simulink model "Demo_Microgrid_OP4510"  (R2017b)
settings: Solver=ode4  StartTime=0.0  StopTime=inf  FixedStep=sim.dt  RelTol=1e-3
values from neighbouring files (symbols this model uses):
  DS001_f0 = 50    [Script_Initialization.m]
  DS001_p0 = 500    [Script_Initialization.m]
  f0_vsi_2 = 50    [Script_Initialization.m]
  kp_vsi_2 = (f0_vsi_2/pmax_vsi_2)*3/1000    (= 7.5e-05)    [Script_Initialization.m]
  kq_vsi_1 = 1e-3    (= 0.001)    [Script_Initialization.m]
  kq_vsi_2 = 1e-3    (= 0.001)    [Script_Initialization.m]
  L_vsi_1 = 2e-3    (= 0.002)    [Script_Initialization.m]
  L_vsi_2 = 2e-3    (= 0.002)    [Script_Initialization.m]
  on_vsi_2 = 1    [Script_Initialization.m]
  p0_vsi_2 = 500    [Script_Initialization.m]
  phi0Deg_vsi_2 = phi0_vsi_2*180/pi    (= 45)    [Script_Initialization.m]
  q0_vsi_2 = 0    [Script_Initialization.m]
  R_vsi_1 = 1e-1    (= 0.1)    [Script_Initialization.m]
  R_vsi_2 = 1e-1    (= 0.1)    [Script_Initialization.m]
  tp_vsi_2 = 100e-3    (= 0.1)    [Script_Initialization.m]
  tq_vsi_1 = 10e-3    (= 0.01)    [Script_Initialization.m]
  tq_vsi_2 = 10e-3    (= 0.01)    [Script_Initialization.m]
  v0_vsi_2 = 340*sqrt(2)    [Script_Initialization.m]
undefined symbols (not defined in the file or in its folder): ld_1, sim, vsi
libraries: powerlib x22, powerlib_meascontrol x5, rtlab x2, xpcrtudplib x2, etargetslib x1, embdlinuxlib x1
settings Model: xpc_rtwmakecfg_data=_xpcnblib__xpcetherlib__xpcether8255xlib__xpcetherGbElib__xpciplib_  Creator=Edwin_Mora  LastModifiedBy=EINS_Admin
settings DebuggingCC: UnconnectedInputMsg=none  UnconnectedOutputMsg=none  UnconnectedLineMsg=none
settings ConfigComp: PSAutoStubLUT=on

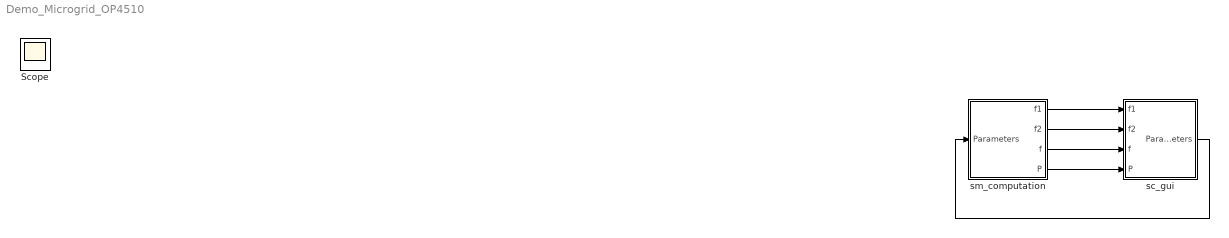
== system Demo_Microgrid_OP4510 ==
  sc_gui : Subsystem
  sm_computation : Subsystem
  Scope : Scope
  wires:
  sm_computation/1(f1) -> sc_gui/1(f1)
  sm_computation/2(f2) -> sc_gui/2(f2)
  sc_gui/1(Parameters) -> sm_computation/1(Parameters)
  sm_computation/3(f) -> sc_gui/3(f)
  sm_computation/4("P ") -> sc_gui/4(P)

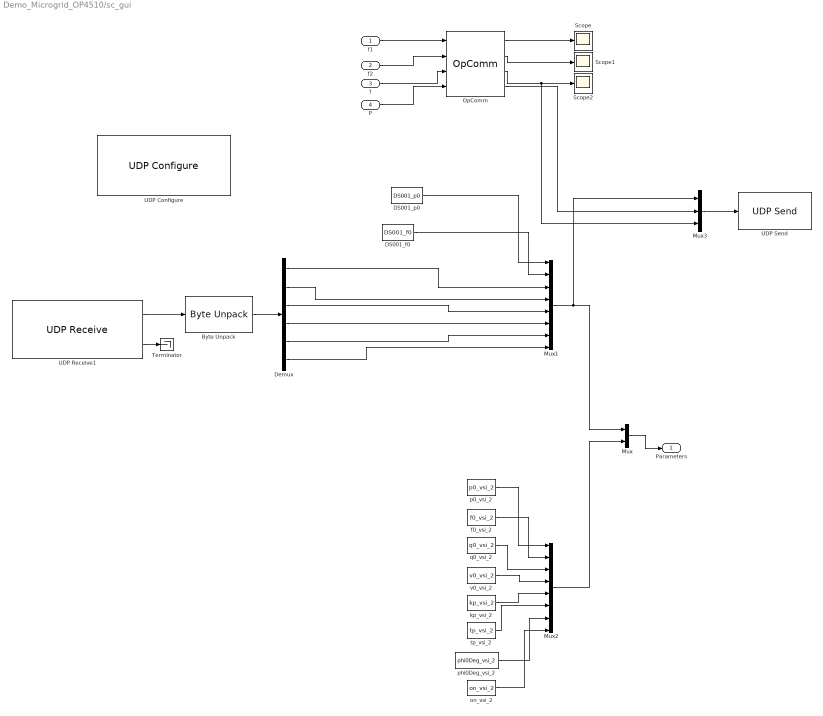
== system Demo_Microgrid_OP4510/sc_gui ==
  f1 : Inport
  f2 : Inport  Port=2
  f : Inport  Port=3
  P : Inport  Port=4
  Byte Unpack : etargetslib/Byte Unpack  dimensions={[6]}  datatypes={'double'}  byteAlign=1
  DS001_f0 : Constant  Value=DS001_f0
  DS001_p0 : Constant  Value=DS001_p0
  Demux : Demux  Outputs=6
  Mux : Mux  Inputs=2
  Mux1 : Mux  Inputs=8
  Mux2 : Mux  Inputs=8
  Mux3 : Mux  Inputs=3
  OpComm : rtlab/OpComm  nbport=4  groupe_acq=1  subsys_rate=0  st=0  Synchronization=on  Interpolation=on  Threshold=1.0  Missed_Data=off  Sim_Time=off  Samples=off  dynSigOut=off  from_console=0  warning_done=off  writeOpCommFile=off  Offset=off
  Scope : Scope
  Scope1 : Scope
  Scope2 : Scope
  Terminator : Terminator
  UDP Configure : xpcrtudplib/UDP Configure  Priority=-1  IpAddress=192.168.1.100  SubnetMask=255.255.255.0  Gateway=0.0.0.0  PciBus=[0]  PciSlot=[6]  PciFunction=0  ID=1  tune=0
      settings: SourceProductName=Simulink Real-Time  SourceProductBaseCode=XP
  UDP Receive1 : xpcrtudplib/UDP Receive  ipAddressVal=192.168.1.100  localPort=8002  rcvWidth=48  rcvFmAny=on  fmAddress=0.0.0.0  maxUDPQueue=8  sampleTime=-1
      settings: SourceProductName=Simulink Real-Time
  UDP Send : embdlinuxlib/UDP Send  remoteURL='192.168.1.11'  remotePort=8001  localURL='255.255.255.255'  localPortSource=Automatically determine  localPort=-1  sampletime=-1  blockPlatform=Raspberry Pi  separateLengthPort=0
      settings: SourceProductName=Simulink Support Package for Raspberry Pi Hardware  SourceProductBaseCode=RASPPI
  f0_vsi_2 : Constant  Value=f0_vsi_2
  kp_vsi_2 : Constant  Value=kp_vsi_2
  on_vsi_2 : Constant  Value=on_vsi_2
  p0_vsi_2 : Constant  Value=p0_vsi_2
  phi0Deg_vsi_2 : Constant  Value=phi0Deg_vsi_2
  q0_vsi_2 : Constant  Value=q0_vsi_2
  tp_vsi_2 : Constant  Value=tp_vsi_2
  v0_vsi_2 : Constant  Value=v0_vsi_2
  Parameters : Outport
  wires:
  f1/1 -> OpComm/1
  OpComm/1 -> Scope/1
  Mux/1 -> Parameters/1
  DS001_p0/1 -> Mux1/1
  DS001_f0/1 -> Mux1/2
  Mux1/1 -> Mux3/1, Mux/1
  f0_vsi_2/1 -> Mux2/2
  p0_vsi_2/1 -> Mux2/1
  on_vsi_2/1 -> Mux2/8
  q0_vsi_2/1 -> Mux2/3
  kp_vsi_2/1 -> Mux2/5
  tp_vsi_2/1 -> Mux2/6
  phi0Deg_vsi_2/1 -> Mux2/7
  v0_vsi_2/1 -> Mux2/4
  Mux2/1 -> Mux/2
  f/1 -> OpComm/3
  OpComm/3 -> Mux3/3, Scope2/1
  f2/1 -> OpComm/2
  OpComm/2 -> Scope1/1
  Mux3/1 -> UDP Send/1
  P/1 -> OpComm/4
  OpComm/4 -> Mux3/2
  UDP Receive1/1 -> Byte Unpack/1
  Demux/1 -> Mux1/3
  Demux/2 -> Mux1/4
  Demux/3 -> Mux1/5
  Demux/4 -> Mux1/6
  Demux/5 -> Mux1/7
  Demux/6 -> Mux1/8
  Byte Unpack/1 -> Demux/1
  UDP Receive1/2 -> Terminator/1

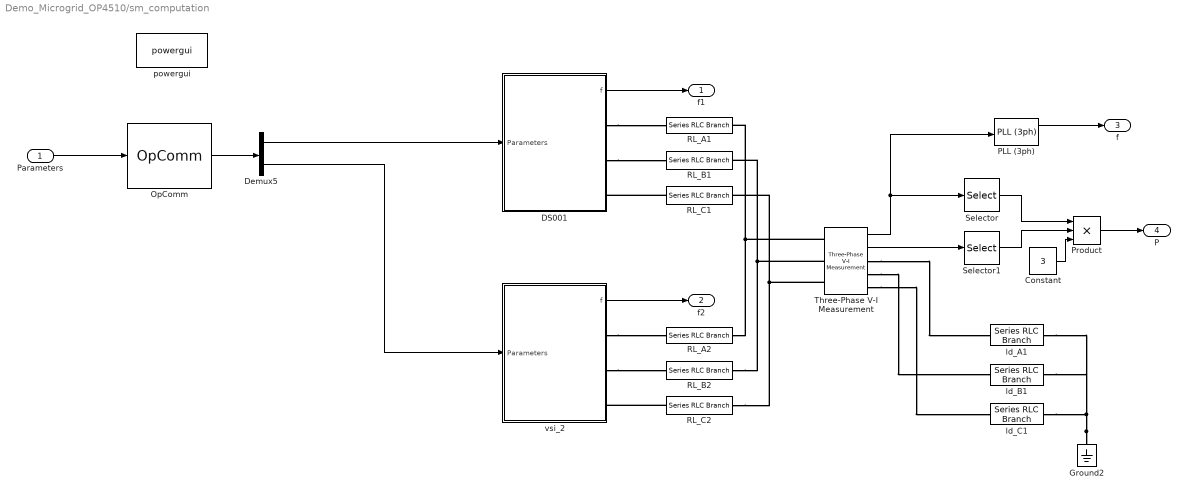
== system Demo_Microgrid_OP4510/sm_computation ==
  Parameters : Inport
  Constant : Constant  Value=3
  DS001 : Subsystem
  Demux5 : Demux  Outputs=2
  Ground2 : powerlib/Elements/Ground  LConnTagsString=a
  OpComm : rtlab/OpComm  nbport=1  groupe_acq=1  subsys_rate=sim.dt  st=0  Synchronization=on  Interpolation=on  Threshold=1.0  Missed_Data=off  Sim_Time=off  Samples=off  dynSigOut=off  from_console=1  warning_done=off  writeOpCommFile=off  Offset=off
  PLL (3ph) : powerlib_meascontrol/PLL/PLL (3ph)  Fmin=45  Par_Init=[0, 50]  ParK=[180, 3200, 1]  TcD=1e-4  MaxRateChangeFreq=12  FilterCutOffFreq=25  Ts=0  AGC=on
  Product : Product  Inputs=3
  RL_A1 : powerlib/Elements/Series RLC Branch  LConnTagsString=__new0  RConnTagsString=__new0  BranchType=RL  Resistance=R_vsi_1  Inductance=L_vsi_1  SetiL0=on  InitialCurrent=0  Capacitance=1e-6  Setx0=off  InitialVoltage=0  Measurements=None
  RL_A2 : powerlib/Elements/Series RLC Branch  LConnTagsString=__new0  RConnTagsString=__new0  BranchType=RL  Resistance=R_vsi_2  Inductance=L_vsi_2  SetiL0=on  InitialCurrent=0  Capacitance=1e-6  Setx0=off  InitialVoltage=0  Measurements=None
  RL_B1 : powerlib/Elements/Series RLC Branch  LConnTagsString=__new0  RConnTagsString=__new0  BranchType=RL  Resistance=R_vsi_1  Inductance=L_vsi_1  SetiL0=on  InitialCurrent=0  Capacitance=1e-6  Setx0=off  InitialVoltage=0  Measurements=None
  RL_B2 : powerlib/Elements/Series RLC Branch  LConnTagsString=__new0  RConnTagsString=__new0  BranchType=RL  Resistance=R_vsi_2  Inductance=L_vsi_2  SetiL0=on  InitialCurrent=0  Capacitance=1e-6  Setx0=off  InitialVoltage=0  Measurements=None
  RL_C1 : powerlib/Elements/Series RLC Branch  LConnTagsString=__new0  RConnTagsString=__new0  BranchType=RL  Resistance=R_vsi_1  Inductance=L_vsi_1  SetiL0=on  InitialCurrent=0  Capacitance=1e-6  Setx0=off  InitialVoltage=0  Measurements=None
  RL_C2 : powerlib/Elements/Series RLC Branch  LConnTagsString=__new0  RConnTagsString=__new0  BranchType=RL  Resistance=R_vsi_2  Inductance=L_vsi_2  SetiL0=on  InitialCurrent=0  Capacitance=1e-6  Setx0=off  InitialVoltage=0  Measurements=None
  Selector : Selector  InputPortWidth=3  IndexOptions=Index vector (dialog)  Indices=[1]  OutputSizes=1
  Selector1 : Selector  InputPortWidth=3  IndexOptions=Index vector (dialog)  Indices=[1]  OutputSizes=1
  Three-Phase V-I Measurement : powerlib/Measurements/Three-Phase V-I Measurement  VoltageMeasurement=phase-to-ground  SetLabelV=off  LabelV=Vabc  Vpu=off  VpuLL=off  CurrentMeasurement=yes  SetLabelI=off  LabelI=Iabc  Ipu=off  Pbase=100e6  Vbase=500e3  OutputType=Complex  PhasorSimulation=off  PSBequivalent=0
  ld_A1 : powerlib/Elements/Series RLC Branch  LConnTagsString=__new0  RConnTagsString=__new0  BranchType=R  Resistance=ld_1.R  Inductance=1e-3  SetiL0=off  InitialCurrent=0  Capacitance=1e-6  Setx0=off  InitialVoltage=0  Measurements=None
  ld_B1 : powerlib/Elements/Series RLC Branch  LConnTagsString=__new0  RConnTagsString=__new0  BranchType=R  Resistance=ld_1.R  Inductance=1e-3  SetiL0=off  InitialCurrent=0  Capacitance=1e-6  Setx0=off  InitialVoltage=0  Measurements=None
  ld_C1 : powerlib/Elements/Series RLC Branch  LConnTagsString=__new0  RConnTagsString=__new0  BranchType=R  Resistance=ld_1.R  Inductance=1e-3  SetiL0=off  InitialCurrent=0  Capacitance=1e-6  Setx0=off  InitialVoltage=0  Measurements=None
  powergui : powerlib/powergui  Priority=1  SimulationMode=Discrete  SampleTime=sim.dt  frequency=50  Iterations=50  frequencyindice=0  Pbase=100e6  ErrMax=1e-4  UnitsV=kV  UnitsW=MW  buscounter=0  FunctionMessages=off  echomessages=off  EnableUseOfTLC=off  CurrentSourceSwitches=off  DisableSnubberDevices=off  DisableRonSwitches=off  DisableVfSwitches=off  DisplayEquations=off  SolverType=Tustin/Backward Euler (TBE)  Interpol=off  ExternalGateDelay=off  methode=off  Ts=100  x0status=blocks  SPID=on  SwTol=0  HookPort=off  RestoreLinks=warning  ResistiveCurrentMeasurement=off  Frange=[0:2:500]  Ylog=off  Xlog=on  ShowGrid=off  save=off  variable=ZData  structure=0  ZoomFFT=off  StartTime=0.0  cycles=1  DisplayStyle=1  fundamental=60  FreqAxis=off  MaxFrequency=1000  frequencyindicesteady=1  RmsSteady=1  display=off
  vsi_2 : Subsystem
  f1 : Outport
  f2 : Outport  Port=2
  f : Outport  Port=3
  "P " : Outport  Port=4
  wires:
  OpComm/1 -> Demux5/1
  Demux5/1 -> DS001/1(Parameters)
  DS001/1(f) -> f1/1
  vsi_2/1(f) -> f2/1
  Demux5/2 -> vsi_2/1(Parameters)
  Parameters/1 -> OpComm/1
  PLL (3ph)/1 -> f/1
  Three-Phase V-I Measurement/1 -> Selector/1, PLL (3ph)/1
  Product/1 -> "P "/1
  Three-Phase V-I Measurement/2 -> Selector1/1
  Selector/1 -> Product/1
  Selector1/1 -> Product/2
  Constant/1 -> Product/3
  connections:
  Ground2/LConn1 -- ld_A1/RConn1 -- ld_B1/RConn1 -- ld_C1/RConn1
  DS001/RConn1 -- RL_A1/LConn1
  DS001/RConn2 -- RL_B1/LConn1
  RL_C1/LConn1 -- DS001/RConn3
  vsi_2/RConn1 -- RL_A2/LConn1
  vsi_2/RConn2 -- RL_B2/LConn1
  RL_C2/LConn1 -- vsi_2/RConn3
  RL_A2/RConn1 -- RL_A1/RConn1 -- Three-Phase V-I Measurement/LConn1
  RL_B2/RConn1 -- Three-Phase V-I Measurement/LConn2 -- RL_B1/RConn1
  RL_C2/RConn1 -- Three-Phase V-I Measurement/LConn3 -- RL_C1/RConn1
  Three-Phase V-I Measurement/RConn1 -- ld_A1/LConn1
  Three-Phase V-I Measurement/RConn2 -- ld_B1/LConn1
  Three-Phase V-I Measurement/RConn3 -- ld_C1/LConn1

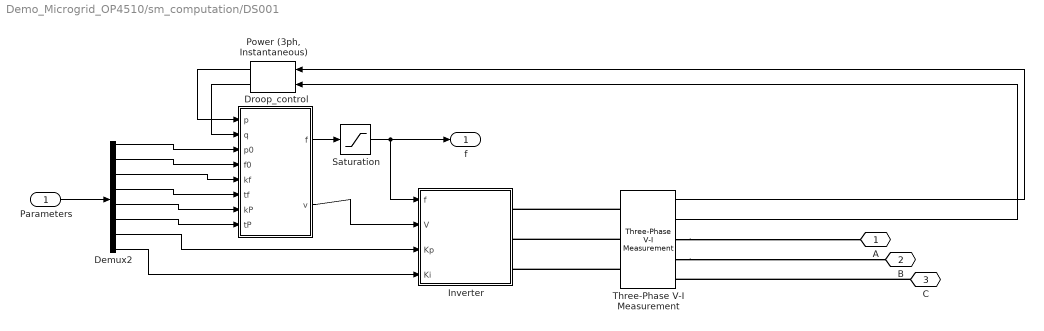
== system Demo_Microgrid_OP4510/sm_computation/DS001 ==
  Parameters : Inport
  Demux2 : Demux  Outputs=8
  Droop_control : Subsystem
  Inverter : Subsystem
  "Power (3ph, Instantaneous)" : powerlib_meascontrol/Measurements/Power (3ph, Instantaneous)
      settings: SourceProductName=Simscape Power Systems
  Saturation : Saturate  UpperLimit=inf  LowerLimit=0
  Three-Phase V-I Measurement : powerlib/Measurements/Three-Phase V-I Measurement  VoltageMeasurement=phase-to-ground  SetLabelV=off  LabelV=Vabc  Vpu=off  VpuLL=off  CurrentMeasurement=yes  SetLabelI=off  LabelI=Iabc  Ipu=off  Pbase=100e6  Vbase=500e3  OutputType=Complex  PhasorSimulation=off  PSBequivalent=0
  A : PMIOPort  Port=1  Side=Right
  B : PMIOPort  Port=2  Side=Right
  C : PMIOPort  Port=3  Side=Right
  f : Outport
  wires:
  Parameters/1 -> Demux2/1
  Demux2/2 -> Droop_control/4(f0)
  Droop_control/2(v) -> Inverter/2(V)
  Demux2/4 -> Droop_control/6(tf)
  Demux2/3 -> Droop_control/5(kf)
  Demux2/6 -> Droop_control/8(tP)
  Demux2/7 -> Inverter/3(Kp)
  Demux2/5 -> Droop_control/7(kP)
  Demux2/1 -> Droop_control/3(p0)
  Saturation/1 -> f/1, Inverter/1(f)
  "Power (3ph, Instantaneous)"/2 -> Droop_control/2(q)
  Three-Phase V-I Measurement/2 -> "Power (3ph, Instantaneous)"/2
  Droop_control/1(f) -> Saturation/1
  "Power (3ph, Instantaneous)"/1 -> Droop_control/1(p)
  Three-Phase V-I Measurement/1 -> "Power (3ph, Instantaneous)"/1
  Demux2/8 -> Inverter/4(Ki)
  connections:
  Three-Phase V-I Measurement/RConn2 -- B/RConn1
  Three-Phase V-I Measurement/LConn1 -- Inverter/RConn1
  Three-Phase V-I Measurement/LConn2 -- Inverter/RConn2
  Three-Phase V-I Measurement/LConn3 -- Inverter/RConn3
  Three-Phase V-I Measurement/RConn1 -- A/RConn1
  C/RConn1 -- Three-Phase V-I Measurement/RConn3

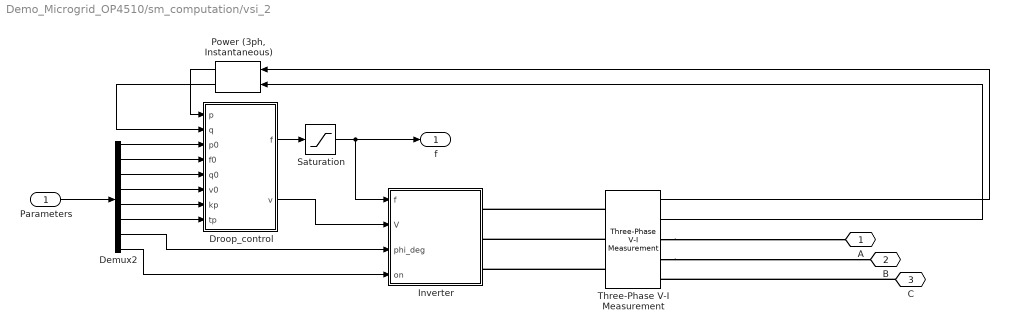
== system Demo_Microgrid_OP4510/sm_computation/vsi_2 ==
  Parameters : Inport
  Demux2 : Demux  Outputs=8
  Droop_control : Subsystem
  Inverter : Subsystem
  "Power (3ph, Instantaneous)" : powerlib_meascontrol/Measurements/Power (3ph, Instantaneous)
      settings: SourceProductName=Simscape Power Systems
  Saturation : Saturate  UpperLimit=inf  LowerLimit=0
  Three-Phase V-I Measurement : powerlib/Measurements/Three-Phase V-I Measurement  VoltageMeasurement=phase-to-ground  SetLabelV=off  LabelV=Vabc  Vpu=off  VpuLL=off  CurrentMeasurement=yes  SetLabelI=off  LabelI=Iabc  Ipu=off  Pbase=100e6  Vbase=500e3  OutputType=Complex  PhasorSimulation=off  PSBequivalent=0
  A : PMIOPort  Port=1  Side=Right
  B : PMIOPort  Port=2  Side=Right
  C : PMIOPort  Port=3  Side=Right
  f : Outport
  wires:
  Demux2/2 -> Droop_control/4(f0)
  Droop_control/2(v) -> Inverter/2(V)
  Demux2/4 -> Droop_control/6(v0)
  Demux2/3 -> Droop_control/5(q0)
  Demux2/6 -> Droop_control/8(tp)
  Parameters/1 -> Demux2/1
  Demux2/5 -> Droop_control/7(kp)
  Demux2/1 -> Droop_control/3(p0)
  Saturation/1 -> f/1, Inverter/1(f)
  "Power (3ph, Instantaneous)"/2 -> Droop_control/2(q)
  Three-Phase V-I Measurement/2 -> "Power (3ph, Instantaneous)"/2
  Droop_control/1(f) -> Saturation/1
  "Power (3ph, Instantaneous)"/1 -> Droop_control/1(p)
  Three-Phase V-I Measurement/1 -> "Power (3ph, Instantaneous)"/1
  Demux2/7 -> Inverter/3(phi_deg)
  Demux2/8 -> Inverter/4(on)
  connections:
  Three-Phase V-I Measurement/RConn2 -- B/RConn1
  Three-Phase V-I Measurement/LConn1 -- Inverter/RConn1
  Three-Phase V-I Measurement/LConn2 -- Inverter/RConn2
  Three-Phase V-I Measurement/LConn3 -- Inverter/RConn3
  Three-Phase V-I Measurement/RConn1 -- A/RConn1
  C/RConn1 -- Three-Phase V-I Measurement/RConn3

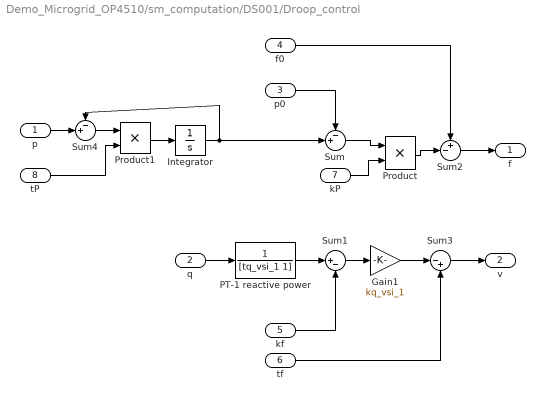
== system Demo_Microgrid_OP4510/sm_computation/DS001/Droop_control ==
  p : Inport
  q : Inport  Port=2
  p0 : Inport  Port=3
  f0 : Inport  Port=4
  kf : Inport  Port=5
  tf : Inport  Port=6
  kP : Inport  Port=7
  tP : Inport  Port=8
  Gain1 : Gain  Gain=kq_vsi_1
  Integrator : Integrator
  PT-1 reactive power : TransferFcn  Denominator=[tq_vsi_1 1]
  Product : Product
  Product1 : Product
  Sum : Sum  Inputs=-+|
  Sum1 : Sum  Inputs=|+-
  Sum2 : Sum  Inputs=+-|
  Sum3 : Sum  Inputs=|-+
  Sum4 : Sum  Inputs=-+|
  f : Outport
  v : Outport  Port=2
  wires:
  Product/1 -> Sum2/2
  Gain1/1 -> Sum3/1
  Sum1/1 -> Gain1/1
  Sum/1 -> Product/1
  Sum3/1 -> v/1
  Sum2/1 -> f/1
  PT-1 reactive power/1 -> Sum1/1
  q/1 -> PT-1 reactive power/1
  p0/1 -> Sum/1
  f0/1 -> Sum2/1
  kf/1 -> Sum1/2
  tf/1 -> Sum3/2
  kP/1 -> Product/2
  p/1 -> Sum4/2
  Sum4/1 -> Product1/1
  Product1/1 -> Integrator/1
  Integrator/1 -> Sum/2, Sum4/1
  tP/1 -> Product1/2

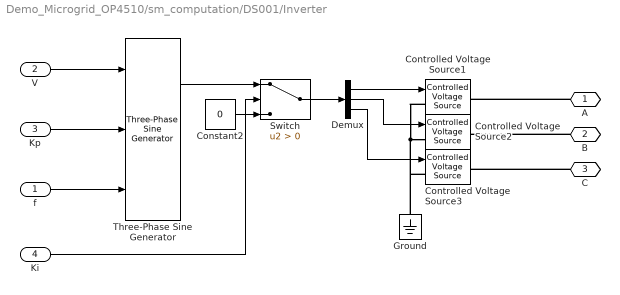
== system Demo_Microgrid_OP4510/sm_computation/DS001/Inverter ==
  f : Inport
  V : Inport  Port=2
  Kp : Inport  Port=3
  Ki : Inport  Port=4
  Constant2 : Constant  Value=0
  Controlled Voltage Source1 : powerlib/Electrical Sources/Controlled Voltage Source  Initialize=off  Source_Type=AC  Amplitude=vsi(1).v0  Phase=vsi(1).phi0*180/pi + 90  Frequency=vsi(1).f0  Measurements=None
  Controlled Voltage Source2 : powerlib/Electrical Sources/Controlled Voltage Source  Initialize=off  Source_Type=AC  Amplitude=vsi(1).v0  Phase=(vsi(1).phi0 - 2*pi/3)*180/pi + 90  Frequency=vsi(1).f0  Measurements=None
  Controlled Voltage Source3 : powerlib/Electrical Sources/Controlled Voltage Source  Initialize=off  Source_Type=AC  Amplitude=vsi(1).v0  Phase=(vsi(1).phi0 - 4*pi/3)*180/pi + 90  Frequency=vsi(1).f0  Measurements=None
  Demux : Demux  Outputs=3
  Ground : powerlib/Elements/Ground  LConnTagsString=a
  Switch : Switch  Criteria=u2 > Threshold
  Three-Phase Sine Generator : powerlib_meascontrol/Pulse & Signal Generators/Three-Phase Sine Generator  Ts=sim.dt
      settings: SourceProductName=Simscape Power Systems  SourceProductBaseCode=PS
  A : PMIOPort  Port=1  Side=Right
  B : PMIOPort  Port=2  Side=Right
  C : PMIOPort  Port=3  Side=Right
  wires:
  Ki/1 -> Switch/2
  f/1 -> Three-Phase Sine Generator/3
  Constant2/1 -> Switch/3
  Switch/1 -> Demux/1
  Three-Phase Sine Generator/1 -> Switch/1
  Demux/1 -> Controlled Voltage Source1/1
  V/1 -> Three-Phase Sine Generator/1
  Demux/3 -> Controlled Voltage Source3/1
  Kp/1 -> Three-Phase Sine Generator/2
  Demux/2 -> Controlled Voltage Source2/1
  connections:
  B/RConn1 -- Controlled Voltage Source2/RConn1
  A/RConn1 -- Controlled Voltage Source1/RConn1
  C/RConn1 -- Controlled Voltage Source3/RConn1
  Controlled Voltage Source1/LConn1 -- Ground/LConn1 -- Controlled Voltage Source3/LConn1 -- Controlled Voltage Source2/LConn1

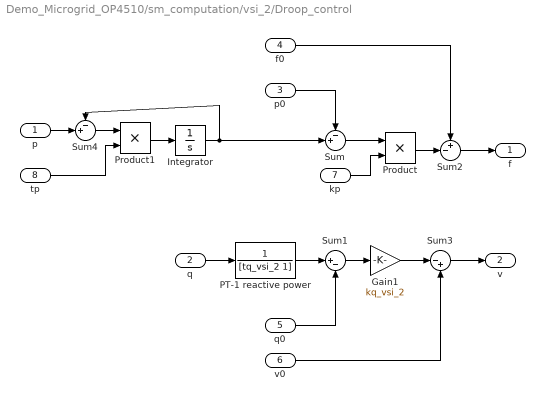
== system Demo_Microgrid_OP4510/sm_computation/vsi_2/Droop_control ==
  p : Inport
  q : Inport  Port=2
  p0 : Inport  Port=3
  f0 : Inport  Port=4
  q0 : Inport  Port=5
  v0 : Inport  Port=6
  kp : Inport  Port=7
  tp : Inport  Port=8
  Gain1 : Gain  Gain=kq_vsi_2
  Integrator : Integrator
  PT-1 reactive power : TransferFcn  Denominator=[tq_vsi_2 1]
  Product : Product
  Product1 : Product
  Sum : Sum  Inputs=-+|
  Sum1 : Sum  Inputs=|+-
  Sum2 : Sum  Inputs=+-|
  Sum3 : Sum  Inputs=|-+
  Sum4 : Sum  Inputs=-+|
  f : Outport
  v : Outport  Port=2
  wires:
  Product/1 -> Sum2/2
  Gain1/1 -> Sum3/1
  Sum1/1 -> Gain1/1
  Sum/1 -> Product/1
  Sum3/1 -> v/1
  Sum2/1 -> f/1
  PT-1 reactive power/1 -> Sum1/1
  q/1 -> PT-1 reactive power/1
  p0/1 -> Sum/1
  f0/1 -> Sum2/1
  q0/1 -> Sum1/2
  v0/1 -> Sum3/2
  kp/1 -> Product/2
  p/1 -> Sum4/2
  Sum4/1 -> Product1/1
  Product1/1 -> Integrator/1
  Integrator/1 -> Sum/2, Sum4/1
  tp/1 -> Product1/2

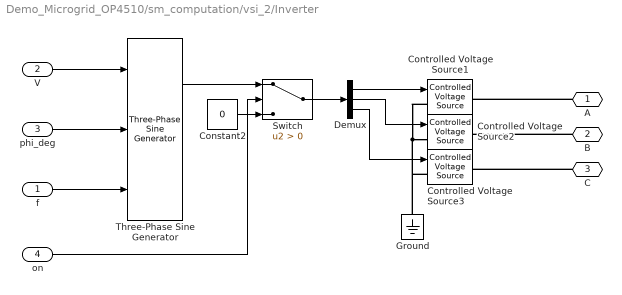
== system Demo_Microgrid_OP4510/sm_computation/vsi_2/Inverter ==
  f : Inport
  V : Inport  Port=2
  phi_deg : Inport  Port=3
  on : Inport  Port=4
  Constant2 : Constant  Value=0
  Controlled Voltage Source1 : powerlib/Electrical Sources/Controlled Voltage Source  Initialize=off  Source_Type=AC  Amplitude=vsi(1).v0  Phase=vsi(1).phi0*180/pi + 90  Frequency=vsi(1).f0  Measurements=None
  Controlled Voltage Source2 : powerlib/Electrical Sources/Controlled Voltage Source  Initialize=off  Source_Type=AC  Amplitude=vsi(1).v0  Phase=(vsi(1).phi0 - 2*pi/3)*180/pi + 90  Frequency=vsi(1).f0  Measurements=None
  Controlled Voltage Source3 : powerlib/Electrical Sources/Controlled Voltage Source  Initialize=off  Source_Type=AC  Amplitude=vsi(1).v0  Phase=(vsi(1).phi0 - 4*pi/3)*180/pi + 90  Frequency=vsi(1).f0  Measurements=None
  Demux : Demux  Outputs=3
  Ground : powerlib/Elements/Ground  LConnTagsString=a
  Switch : Switch  Criteria=u2 > Threshold
  Three-Phase Sine Generator : powerlib_meascontrol/Pulse & Signal Generators/Three-Phase Sine Generator  Ts=sim.dt
      settings: SourceProductName=Simscape Power Systems  SourceProductBaseCode=PS
  A : PMIOPort  Port=1  Side=Right
  B : PMIOPort  Port=2  Side=Right
  C : PMIOPort  Port=3  Side=Right
  wires:
  on/1 -> Switch/2
  f/1 -> Three-Phase Sine Generator/3
  Constant2/1 -> Switch/3
  Switch/1 -> Demux/1
  Three-Phase Sine Generator/1 -> Switch/1
  Demux/1 -> Controlled Voltage Source1/1
  V/1 -> Three-Phase Sine Generator/1
  Demux/3 -> Controlled Voltage Source3/1
  phi_deg/1 -> Three-Phase Sine Generator/2
  Demux/2 -> Controlled Voltage Source2/1
  connections:
  B/RConn1 -- Controlled Voltage Source2/RConn1
  A/RConn1 -- Controlled Voltage Source1/RConn1
  C/RConn1 -- Controlled Voltage Source3/RConn1
  Controlled Voltage Source1/LConn1 -- Ground/LConn1 -- Controlled Voltage Source3/LConn1 -- Controlled Voltage Source2/LConn1
